simulink model "SimModel"  (R2024a)
settings: Solver=FixedStepAuto  StartTime=0.0  StopTime=3  FixedStep=dt  RelTol=1e-3
values from neighbouring files (symbols this model uses):
  amp = 200    [initialize.m]
  B = [0; 0; 1/L]    [LQR.m]    (also in initialize.m = 5.09e-05; transfer_function.m = 5.09e-05)
  cpr = 360000    [initialize.m]
  dt = 0.00001    (= 1e-05)    [initialize.m]
  end_freq = 20    [initialize.m]
  J = 2.28e-7    (= 2.28e-07)    [LQR.m]    (also in initialize.m; transfer_function.m)
  K_e = 17.8e-3    (= 0.0178)    [LQR.m]    (also in initialize.m; transfer_function.m)
  K_t = 17.8e-3    (= 0.0178)    [LQR.m]    (also in initialize.m; transfer_function.m)
  Kd_pos = 0.43    [calculate_loss.m]    (also in initialize.m = 0.0134; optimize_cascade_pid_outter.m = parameters(3); transfer_function.m = 0.0134)
  Kd_vel = 0.000005    (= 5e-06)    [calculate_loss.m]    (also in initialize.m; optimize_cascade_pid_inner.m = parameters(3); transfer_function.m)
  Ki_pos = 0.2694    [calculate_loss.m]    (also in initialize.m; optimize_cascade_pid_outter.m = parameters(2); transfer_function.m)
  Ki_vel = 0.67    [calculate_loss.m]    (also in initialize.m; optimize_cascade_pid_inner.m = parameters(2); transfer_function.m)
  Kp_pos = 140    [calculate_loss.m]    (also in initialize.m; optimize_cascade_pid_outter.m = parameters(1); transfer_function.m = 135)
  Kp_vel = 0.6    [calculate_loss.m]    (also in initialize.m; optimize_cascade_pid_inner.m = parameters(1); transfer_function.m = 0.61)
  L = 0.411e-3    (= 0.000411)    [LQR.m]    (also in initialize.m; transfer_function.m)
  R = 10    [LQR.m]    (also in initialize.m = 6.23; transfer_function.m = 6.23)
  signal_switch = 1    [initialize.m]
  start_freq = 1    [initialize.m]
  start_time = 1    [initialize.m]
  time_range = 200    [initialize.m]
libraries: simulink_extras x1
settings Model: Creator=dogu1  LastModifiedBy=HP
settings OptimizationCC: ReuseModelBlockBuffer=off
settings RTWCC: GPUComputeCapability=3.5

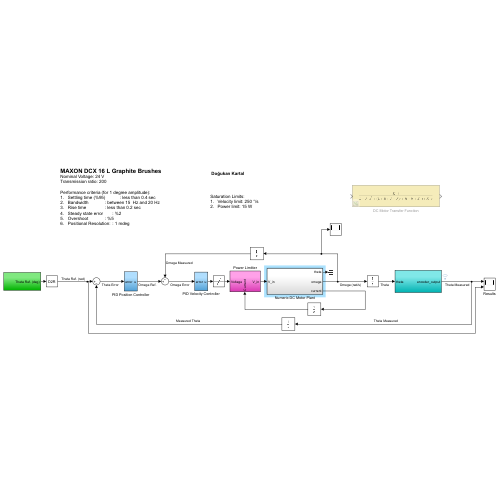
[thumbnail: Simulink's stored preview of the top-level diagram]
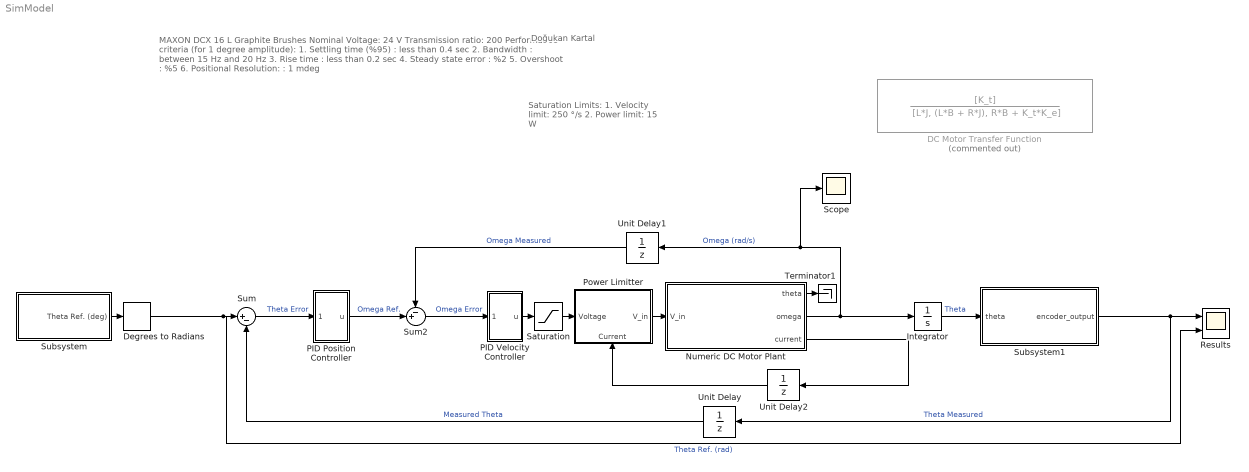
== system SimModel ==
  note: Saturation Limits:
      | 1. Velocity limit: 250 °/s
      | 2. Power limit: 15 W
  note: MAXON DCX 16 L Graphite Brushes
      | Nominal Voltage: 24 V
      | Transmission ratio: 200
      |
      | Performance criteria (for 1 degree amplitude):
      | 1. Settling time (%95) : less than 0.4 sec
      | 2. Bandwidth : between 15 Hz and 20 Hz
      | 3. Rise time : less than 0.2 sec
      | 4. Steady state error : %2
      | 5. Overshoot : %5
      | 6. Positional Resolution: : 1 mdeg
  note: Doğukan Kartal
  DC Motor Transfer Function : TransferFcn  Commented=on  Numerator=[K_t]  Denominator=[L*J, (L*B + R*J), R*B + K_t*K_e]
  Degrees to Radians : simulink_extras/Transformations/Degrees to Radians
  Integrator : Integrator
  Numeric DC Motor Plant : Subsystem
  PID Position Controller : Subsystem
  PID Velocity Controller : Subsystem
  Power Limitter : Subsystem
      settings: PortSchema="{\"entries\":[{\"content\":{\"sides\":[{\"content\":{\"connectorIds\":[\"In1\"]},\"type\":\"ConnectorPlacement.EquallySpacedRectSide\",\"uuid\":\"0eeb06f6-9815-4848-984a-49d97fe300a8\"},{\"content\":{\"connectorIds\":[\"Out1\"],\"side\":\"RIGHT\"},\"type\":\"ConnectorPlacement.EquallySpacedRectSide\",\"uuid\":\"7a8b407b-a98a-4788-978f-1411a8c2a655\"},{\"content\":{\"side\":\"TOP\"},\"type\":\"ConnectorPlacement.EquallySpacedRectSide\",\"uuid\":\"95c101ac-3588-46e5-9809-7b6d81ee47be\"},{\"content\":{\"connectorIds\":[\"In2\"],\"side\":\"BOTTOM\"},\"type\":\"ConnectorPlacement.EquallySpacedRectSide\",\"uuid\":\"0f0efbe0-a92a-4c17-a6bf-7c528c3d3295\"}]},\"type\":\"ConnectorPlacement.EquallySpacedConnector\",\"uuid\":\"e2d8baa3-2ad4-48eb-beae-21b8365f5f81\"}],\"packageUris\":[\"http://schema.mathworks.com/mf0/Connector/R2020b\"],\"version\":\"1.0\"}"
  Results : Scope  NumInputPorts=2
  Saturation : Saturate  UpperLimit=24  LowerLimit=-24
  Scope : Scope
  Subsystem : Subsystem
  Subsystem1 : Subsystem
  Sum : Sum  Inputs=|+-
  Sum2 : Sum  Inputs=-+|
  Terminator1 : Terminator
  Unit Delay : UnitDelay  SampleTime=-1  HasFrameUpgradeWarning=on
  Unit Delay1 : UnitDelay  SampleTime=-1  HasFrameUpgradeWarning=on
  Unit Delay2 : UnitDelay  SampleTime=-1  HasFrameUpgradeWarning=on
  wires:
  Unit Delay/1 -> Sum/2  "Measured Theta"
  Subsystem1/1(encoder_output) -> Results/1, Unit Delay/1  "Theta Measured"
  Sum2/1 -> PID Velocity Controller/1(error)  "Omega Error"
  Unit Delay1/1 -> Sum2/1  "Omega Measured"
  Degrees to Radians/1 -> Sum/1, Results/2  "Theta Ref. (rad)"
  Sum/1 -> PID Position Controller/1(error)  "Theta Error"
  PID Position Controller/1(u) -> Sum2/2  "Omega Ref."
  Numeric DC Motor Plant/2(omega) -> Integrator/1, Unit Delay1/1, Scope/1  "Omega (rad/s)"
  Numeric DC Motor Plant/3(current) -> Unit Delay2/1
  PID Velocity Controller/1(u) -> Saturation/1
  Integrator/1 -> Subsystem1/1(theta)  "Theta"
  Subsystem/1(Theta Ref. (deg)) -> Degrees to Radians/1
  Saturation/1 -> Power Limitter/1(Voltage)
  Numeric DC Motor Plant/1(theta) -> Terminator1/1
  Unit Delay2/1 -> Power Limitter/2(Current)
  Power Limitter/1(V_in) -> Numeric DC Motor Plant/1(V_in)

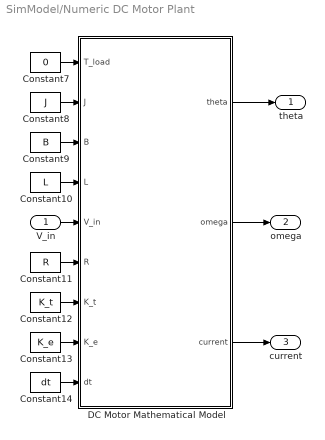
== system SimModel/Numeric DC Motor Plant ==
  V_in : Inport
  Constant10 : Constant  Value=L
  Constant11 : Constant  Value=R
  Constant12 : Constant  Value=K_t
  Constant13 : Constant  Value=K_e
  Constant14 : Constant  Value=dt
  Constant7 : Constant  Value=0
  Constant8 : Constant  Value=J
  Constant9 : Constant  Value=B
  DC Motor Mathematical Model : MATLAB Function  TreatAsAtomicUnit=on
  theta : Outport
  omega : Outport  Port=2
  current : Outport  Port=3
  wires:
  Constant12/1 -> DC Motor Mathematical Model/7(K_t)
  Constant10/1 -> DC Motor Mathematical Model/4(L)
  Constant7/1 -> DC Motor Mathematical Model/1(T_load)
  Constant14/1 -> DC Motor Mathematical Model/9(dt)
  Constant8/1 -> DC Motor Mathematical Model/2(J)
  Constant13/1 -> DC Motor Mathematical Model/8(K_e)
  Constant11/1 -> DC Motor Mathematical Model/6(R)
  Constant9/1 -> DC Motor Mathematical Model/3(B)
  DC Motor Mathematical Model/3(current) -> current/1
  DC Motor Mathematical Model/2(omega) -> omega/1
  DC Motor Mathematical Model/1(theta) -> theta/1
  V_in/1 -> DC Motor Mathematical Model/5(V_in)

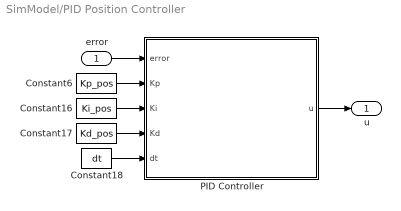
== system SimModel/PID Position Controller ==
  error : Inport
  Constant16 : Constant  Value=Ki_pos
  Constant17 : Constant  Value=Kd_pos
  Constant18 : Constant  Value=dt
  Constant6 : Constant  Value=Kp_pos
  PID Controller : MATLAB Function  TreatAsAtomicUnit=on
  u : Outport
  wires:
  PID Controller/1(u) -> u/1
  Constant16/1 -> PID Controller/3(Ki)
  Constant17/1 -> PID Controller/4(Kd)
  Constant18/1 -> PID Controller/5(dt)
  Constant6/1 -> PID Controller/2(Kp)
  error/1 -> PID Controller/1(error)

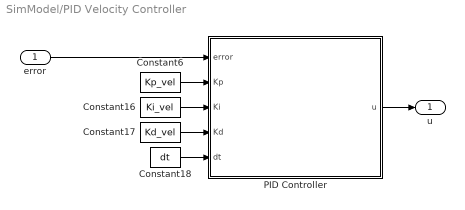
== system SimModel/PID Velocity Controller ==
  error : Inport
  Constant16 : Constant  Value=Ki_vel
  Constant17 : Constant  Value=Kd_vel
  Constant18 : Constant  Value=dt
  Constant6 : Constant  Value=Kp_vel
  PID Controller : MATLAB Function  TreatAsAtomicUnit=on
  u : Outport
  wires:
  error/1 -> PID Controller/1(error)
  Constant6/1 -> PID Controller/2(Kp)
  Constant18/1 -> PID Controller/5(dt)
  Constant17/1 -> PID Controller/4(Kd)
  Constant16/1 -> PID Controller/3(Ki)
  PID Controller/1(u) -> u/1

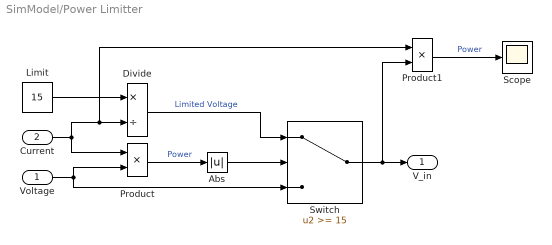
== system SimModel/Power Limitter ==
  Voltage : Inport
  Current : Inport  Port=2
  Abs : Abs  SaturateOnIntegerOverflow=off
  Divide : Product  Inputs=*/
  Limit : Constant  Value=15
  Product : Product
  Product1 : Product
  Scope : Scope
  Switch : Switch  Threshold=15  SaturateOnIntegerOverflow=off  InputSameDT=off
  V_in : Outport
  wires:
  Current/1 -> Product1/1, Divide/2, Product/1
  Product/1 -> Abs/1  "Power"
  Switch/1 -> Product1/2, V_in/1
  Divide/1 -> Switch/1  "Limited Voltage"
  Voltage/1 -> Switch/3, Product/2
  Limit/1 -> Divide/1
  Product1/1 -> Scope/1  "Power"
  Abs/1 -> Switch/2

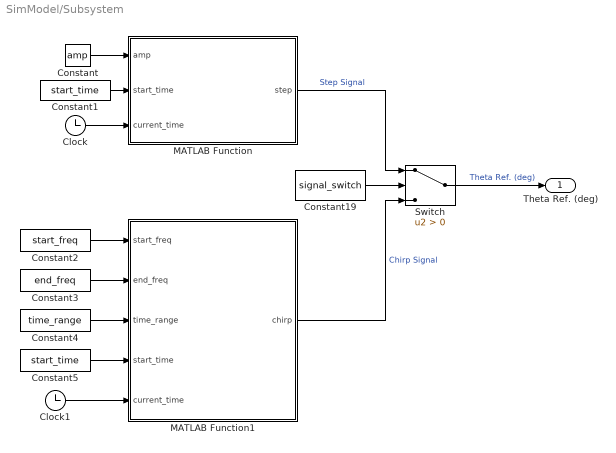
== system SimModel/Subsystem ==
  Clock : Clock
  Clock1 : Clock
  Constant : Constant  Value=amp
  Constant1 : Constant  Value=start_time
  Constant19 : Constant  Value=signal_switch
  Constant2 : Constant  Value=start_freq
  Constant3 : Constant  Value=end_freq
  Constant4 : Constant  Value=time_range
  Constant5 : Constant  Value=start_time
  MATLAB Function : MATLAB Function  TreatAsAtomicUnit=on
  MATLAB Function1 : MATLAB Function  TreatAsAtomicUnit=on
  Switch : Switch  Criteria=u2 > Threshold  SaturateOnIntegerOverflow=off  InputSameDT=off
  Theta Ref. (deg) : Outport
  wires:
  MATLAB Function/1(step) -> Switch/1  "Step Signal"
  Constant2/1 -> MATLAB Function1/1(start_freq)
  MATLAB Function1/1(chirp) -> Switch/3  "Chirp Signal"
  Clock1/1 -> MATLAB Function1/5(current_time)
  Clock/1 -> MATLAB Function/3(current_time)
  Constant19/1 -> Switch/2
  Switch/1 -> Theta Ref. (deg)/1  "Theta Ref. (deg)"
  Constant/1 -> MATLAB Function/1(amp)
  Constant3/1 -> MATLAB Function1/2(end_freq)
  Constant4/1 -> MATLAB Function1/3(time_range)
  Constant1/1 -> MATLAB Function/2(start_time)
  Constant5/1 -> MATLAB Function1/4(start_time)

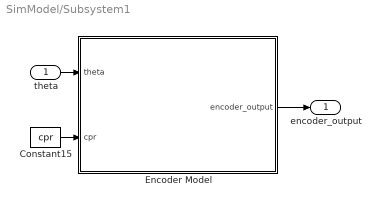
== system SimModel/Subsystem1 ==
  theta : Inport
  Constant15 : Constant  Value=cpr
  Encoder Model : MATLAB Function  TreatAsAtomicUnit=on
  encoder_output : Outport
  wires:
  theta/1 -> Encoder Model/1(theta)
  Constant15/1 -> Encoder Model/2(cpr)
  Encoder Model/1(encoder_output) -> encoder_output/1

== matlab function SimModel/Subsystem/MATLAB Function1 ==
  data: start_freq input; chirp output; end_freq input; time_range input; start_time input; current_time input
function chirp  = generate_chirp(start_freq, end_freq, time_range, start_time, current_time)
    
    if current_time >= start_time && current_time <= time_range
        k = (end_freq - start_freq) / time_range;
        chirp = sin(2 * pi * (start_freq * current_time + 0.5 * k * current_time^2));
    else
        chirp = 0;
    end
end

== matlab function SimModel/Subsystem/MATLAB Function ==
  data: amp input; step output; start_time input; current_time input
function step  = generate_step(amp, start_time, current_time)
    if current_time >= start_time
        step = amp;
    else
        step = 0;
    end
end

== matlab function SimModel/Numeric DC Motor Plant/DC Motor Mathematical Model ==
  settings: updateMethod=DISCRETE
  data: T_load input; J input; B input; L input; V_in input; theta output; R input; K_t input; K_e input; dt input; omega output; current output
function [theta, omega, current] = DCmotor(T_load, J, B, L, V_in, R, K_t, K_e, dt)
    % V_in: Input Voltage (V) {24}
    % T_load: Load torque (Nm)
    % J: Moment of Inertia (kg.m^2) {2.28 x 10^(-7)}
    % B: Viscous Damping Coefficient (Nm.s/rad) {5.09 x 10^(-5)}
    % L: Inductance (H) {0.411 x 10^(-3)}
    % R: Resistance (Ohm) {6.23}
    % K_t: Torque Constant (Nm/A) {17.8 x 10^(-3)}
    % K_e: Back EMF Constant (V/(rad/s)) {0.0178}
    % dt: Time step (s)

    persistent prev_theta prev_omega prev_current

    if isempty(prev_theta)
        prev_theta = 0;
        prev_omega = 0;
        prev_current = 0;
    end

    %Electrical Equation
    dI_dt = (V_in - K_e * prev_omega - R * prev_current) / L;
    current = prev_current + dI_dt * dt;

    %Mechanical Equation
    domega_dt = (K_t * current - B * prev_omega - T_load) / J;


    omega = prev_omega + domega_dt * dt;

    

    %Update
    theta = prev_theta + prev_omega * dt;
    prev_theta = theta;
    prev_omega = omega;
    prev_current = current;

end

== matlab function SimModel/Subsystem1/Encoder Model ==
  data: theta input; encoder_output output; cpr input
function encoder_output  = encoder(theta, cpr)
    count = round(theta * (cpr / (2 * pi)));
    encoder_output = count * (2 * pi / cpr);
end

== matlab function SimModel/PID Velocity Controller/PID Controller ==
  data: error input; u output; Kp input; Ki input; Kd input; dt input
function u = PID(error, Kp, Ki, Kd, dt)
        
    persistent prev_error error_sum
    
    if isempty(prev_error)
        prev_error = 0;
        error_sum = 0;
    end
    
    %Proportional
    P = Kp * error;
    
    %Integral
    error_sum = error_sum + error * dt;
    I = Ki * error_sum;
    
    %Derivative
    D = Kd * (error - prev_error) / dt;
    
    %Control Signal
    u = P + I + D;
    
    %Update of Previous Error
    prev_error = error;

end

== matlab function SimModel/PID Position Controller/PID Controller ==
  settings: updateMethod=DISCRETE
  data: error input; u output; Kp input; Ki input; Kd input; dt input
function u = PID(error, Kp, Ki, Kd, dt)
        
    persistent prev_error error_sum
    
    if isempty(prev_error)
        prev_error = 0;
        error_sum = 0;
    end
    
    %Proportional
    P = Kp * error;
    
    %Integral
    error_sum = error_sum + error * dt;
    I = Ki * error_sum;
    
    %Derivative
    D = Kd * (error - prev_error) / dt;
    
    %Control Signal
    u = P + I + D;
    
    %Update of Previous Error
    prev_error = error;

end
